simulink subsystem "rss_ElecAgCalcNeed"  (R2023a)
settings: Solver=VariableStepAuto  StartTime=0.0  StopTime=10.0  RelTol=1e-3
libraries: lib_conversion x1, lib_configurable_parameter x1
settings Model: Creator=xiaoqiang.yuan  LastModifiedBy=xiaoqiang.yuan

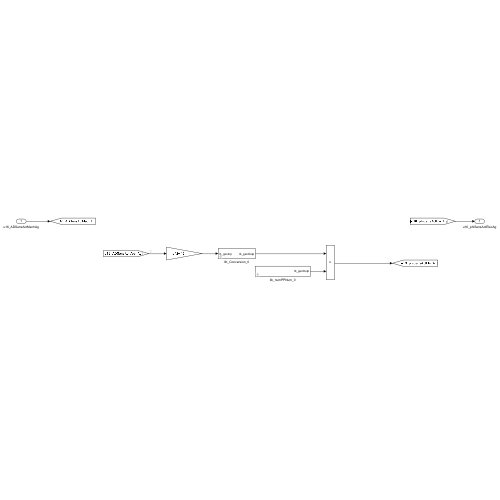
[thumbnail: Simulink's stored preview of the top-level diagram]
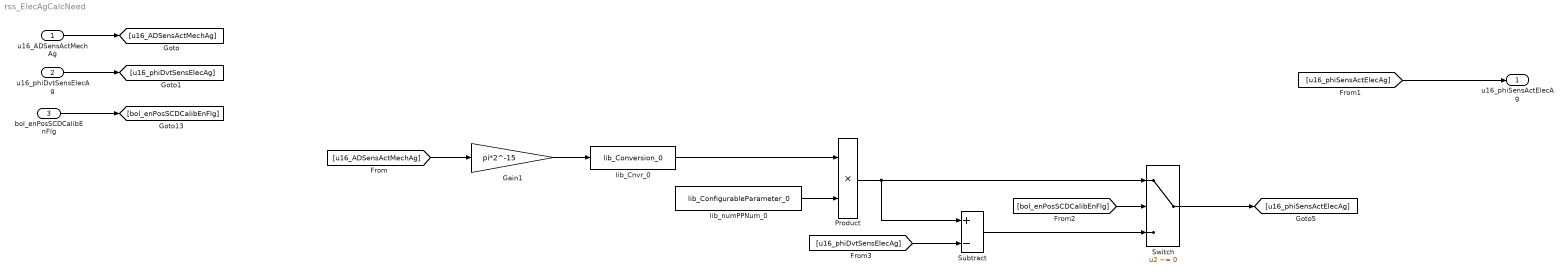
== system rss_ElecAgCalcNeed ==
  u16_ADSensActMechAg : Inport  OutDataTypeStr=uint16
  u16_phiDvtSensElecAg : Inport  Port=2  OutDataTypeStr=dt_RadAng_u16r15b0
  bol_enPosSCDCalibEnFlg : Inport  Port=3  OutDataTypeStr=boolean
  Gain1 : Gain  Gain=pi*2^-15  OutDataTypeStr=Inherit: Inherit via back propagation  RndMeth=Simplest
  Product : Product  InitFcn=|  RndMeth=Simplest  OutDataTypeStr=Inherit: Same as first input
      | Simulink.suppressDiagnostic(gcb,...
      | 'SimulinkFixedPoint:util:Overflowoccurred');
  Subtract : Sum  Inputs=+-  OutDataTypeStr=Inherit: Same as first input
  Switch : Switch  Criteria=u2 ~= 0  SaturateOnIntegerOverflow=off  InputSameDT=off
  lib_Cnvr_0 : lib_conversion/lib_Conversion_0  lb_parDataType=dt_RadAng_u16r15b0  lb_parOutpMaxVal=[]  lb_parOutpMinVal=[]  lb_parSatFlag=off
  lib_numPPNum_0 : lib_configurable_parameter/lib_ConfigurableParameter_0  lb_parCnfgPar=Gu8_numPPNum_C  lb_parDataType=Inherit: Inherit from 'Constant value'  lb_parUpLim=Cdbl_numPPNumMaxVal  lb_parLowLim=Cdbl_numPPNumMinVal
  u16_phiSensActElecAg : Outport  OutDataTypeStr=dt_RadAng_u16r15b0
  wires:
  [u16_ADSensActMechAg] -> Gain1/1
  u16_ADSensActMechAg/1 -> [u16_ADSensActMechAg]
  Gain1/1 -> lib_Cnvr_0/1
  lib_Cnvr_0/1 -> Product/1
  lib_numPPNum_0/1 -> Product/2
  [u16_phiSensActElecAg] -> u16_phiSensActElecAg/1
  bol_enPosSCDCalibEnFlg/1 -> [bol_enPosSCDCalibEnFlg]
  u16_phiDvtSensElecAg/1 -> [u16_phiDvtSensElecAg]
  Product/1 -> Switch/1, Subtract/1
  [bol_enPosSCDCalibEnFlg] -> Switch/2
  Subtract/1 -> Switch/3
  Switch/1 -> [u16_phiSensActElecAg]
  [u16_phiDvtSensElecAg] -> Subtract/2
